simulink model "preLookupTestGen18"  (R2017b)
settings: Solver=FixedStepDiscrete  StartTime=0.0  StopTime=10.0  RelTol=1e-3
settings Model: Creator=ktrinh  LastModifiedBy=ktrinh
settings DebuggingCC: ParameterOverflowMsg=none

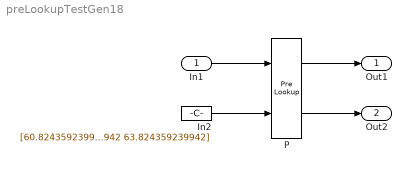
== system preLookupTestGen18 ==
  In1 : Inport  OutDataTypeStr=double  PortDimensions=3
  In2 : Constant  Value=[60.824359239942 62.324359239942 63.824359239942]
  P : PreLookup  BreakpointsDataSource=Input port  BreakpointsData=[10:10:110]  IndexSearchMethod=Linear search  BeginIndexSearchUsingPreviousIndexResult=on  BreakpointDataTypeStr=int32  IndexDataTypeStr=int8  FractionDataTypeStr=double  RndMeth=Round
      settings: InputPortMap=u0,p1
  Out1 : Outport
  Out2 : Outport  Port=2
  wires:
  In1/1 -> P/1
  In2/1 -> P/2
  P/1 -> Out1/1
  P/2 -> Out2/1
